simulink model "model_main_test"  (R2020b)
settings: configuration reference "Configuration" (kept outside this file)
settings Model: Creator=dogukan  LastModifiedBy=dogukan
settings ConfigSetRef: SourceName=Configuration  SourceLocation=Base Workspace

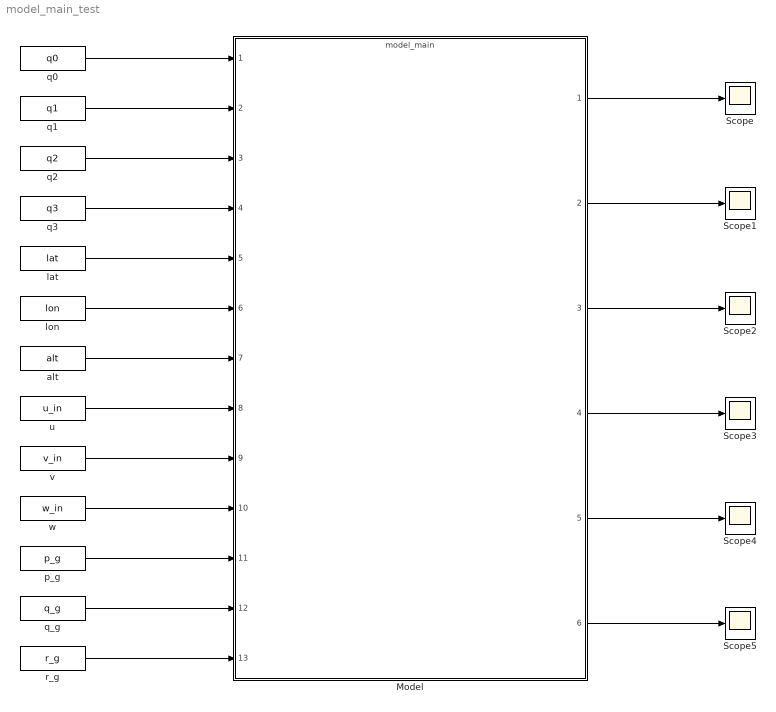
== system model_main_test ==
  Model : ModelReference  ModelNameDialog=model_main.slx  SimulationMode=Normal  ModelReferenceVersion=1.442
  Scope{,1..5} (6 alike) : Scope
  alt : FromWorkspace  VariableName=alt
  lat : FromWorkspace  VariableName=lat
  lon : FromWorkspace  VariableName=lon
  p_g : FromWorkspace  VariableName=p_g
  q0 : FromWorkspace  VariableName=q0
  q1 : FromWorkspace  VariableName=q1
  q2 : FromWorkspace  VariableName=q2
  q3 : FromWorkspace  VariableName=q3
  q_g : FromWorkspace  VariableName=q_g
  r_g : FromWorkspace  VariableName=r_g
  u : FromWorkspace  VariableName=u_in
  v : FromWorkspace  VariableName=v_in
  w : FromWorkspace  VariableName=w_in
  wires:
  Model/1 -> Scope/1
  Model/3 -> Scope2/1
  Model/2 -> Scope1/1
  alt/1 -> Model/7
  lat/1 -> Model/5
  lon/1 -> Model/6
  q0/1 -> Model/1
  q2/1 -> Model/3
  q1/1 -> Model/2
  q3/1 -> Model/4
  u/1 -> Model/8
  v/1 -> Model/9
  w/1 -> Model/10
  q_g/1 -> Model/12
  p_g/1 -> Model/11
  r_g/1 -> Model/13
  Model/4 -> Scope3/1
  Model/5 -> Scope4/1
  Model/6 -> Scope5/1
